simulink model "greenLed"  (R2018b)
settings: Solver=FixedStepAuto  StartTime=0.0  StopTime=inf  RelTol=1e-3  EnableMultiTasking=on
settings Model: SimulationMode=external  Creator=dskiee  LastModifiedBy=my3197
settings SolverCC: PositivePriorityOrder=on
settings OptimizationCC: EnhancedBackFolding=on  PassReuseOutputArgsAs=Individual arguments  MaxStackSize=64  OptimizeBlockOrder=speed  DifferentSizesBufferReuse=on  OptimizationCustomize=off
settings DebuggingCC: ParameterTunabilityLossMsg=error
settings HardwareCC: ProdBitPerPointer=32  ProdBitPerSizeT=32  ProdBitPerPtrDiffT=32  ProdLargestAtomicInteger=Long  ProdLargestAtomicFloat=Double  ProdWordSize=32  ProdHWDeviceType=ARM Compatible->ARM Cortex
settings SFSimCC: MATLABDynamicMemAlloc=off
settings RTWCC: SystemTargetFile=ert.tlc  HardwareBoard=Xilinx Zynq-7000 based board  TLCOptions="-aInlineSetEventsForThisBaseRateFcn=TLC_FALSE -aSuppressMultiTaskScheduler=TLC_FALSE  -aRateBasedStepFcn=0"  TemplateMakefile=ert_default_tmf  GenerateReport=on  Toolchain=Linaro AArch32 Linux v6.3.1  IncludeHyperlinkInReport=on  LaunchReport=on  GenerateTraceInfo=on  GenerateTraceReport=on  GenerateTraceReportSl=on  GenerateTraceReportSf=on  GenerateTraceReportEml=on
settings CodeAppCC: ForceParamTrailComments=on  IgnoreCustomStorageClasses=off  OperatorAnnotations=on  SimulinkDataObjDesc=on  SFDataObjDesc=on  InsertBlockDesc=on
settings ERTTargetCC: SupportNonInlinedSFcns=on

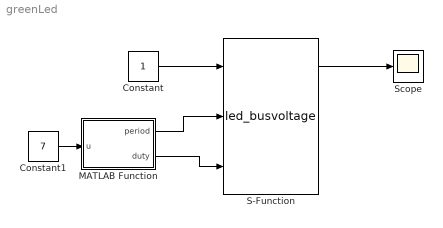
== system greenLed ==
  Constant : Constant
  Constant1 : Constant  Value=7
  MATLAB Function : MATLAB Function  TreatAsAtomicUnit=on
  S-Function : S-Function  FunctionName=led_busvoltage  SFunctionDeploymentMode=off  EnableBusSupport=off
  Scope : Scope
  wires:
  S-Function/1 -> Scope/1
  Constant/1 -> S-Function/1
  MATLAB Function/1(period) -> S-Function/2
  MATLAB Function/2(duty) -> S-Function/3
  Constant1/1 -> MATLAB Function/1(u)

== matlab function greenLed/MATLAB Function ==
  data: u input; period output; duty output
function [period,duty]= fcn(u)

if u > 7.4
    period = 50000000;
    duty = 50000000;
elseif u <=7.4 && u > 6.8
    period = 50000000;
    duty = 25000000;
elseif u <= 6.8
    period = 5000000;
    duty = 2500000;
else
    period = 0;
    duty = 0;
end
